simulink model "A3_2_InvKin_testing"  (R2023a)
settings: Solver=VariableStepAuto  StartTime=0.0  StopTime=10.0  RelTol=1e-3
values from neighbouring files (symbols this model uses):
  params = [l2 l3]    [A3_1_init_VorKin.m]    (also in A3_2_init_InvKin.m; init_InvKin.m)
settings Model: Creator=Flo  LastModifiedBy=Flo

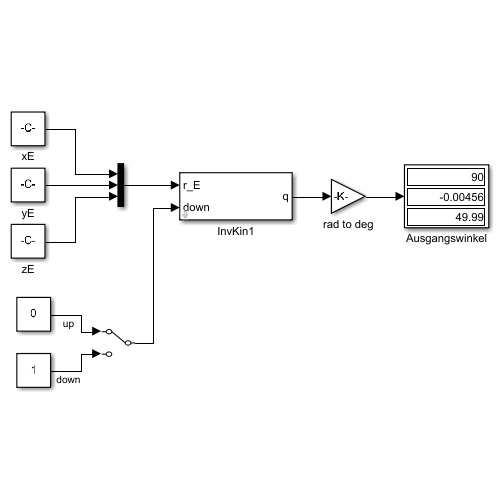
[thumbnail: Simulink's stored preview of the top-level diagram]
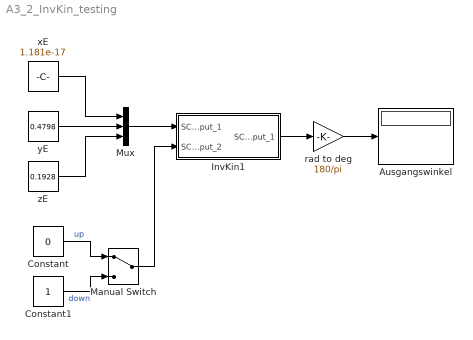
== system A3_2_InvKin_testing ==
  Ausgangswinkel : Display
  Constant : Constant  Value=0
  Constant1 : Constant
  InvKin1 : Subsystem  mask{SC_param_0=params}
      mask prompts: SC_param_0 "params"
      mask Display:
      | port_label('input', 1, 'r_E');
      | port_label('input', 2, 'down');
      | port_label('output', 1, 'q');
  Manual Switch : ManualSwitch
  Mux : Mux  Inputs=3
  rad to deg : Gain  Gain=180/pi
  xE : Constant  Value=1.181e-17
  yE : Constant  Value=0.4798
  zE : Constant  Value=0.1928
  wires:
  zE/1 -> Mux/3
  xE/1 -> Mux/1
  yE/1 -> Mux/2
  Mux/1 -> InvKin1/1(SC_input_1)
  Manual Switch/1 -> InvKin1/2(SC_input_2)
  Constant1/1 -> Manual Switch/2  "down"
  Constant/1 -> Manual Switch/1  "up"
  InvKin1/1(SC_output_1) -> rad to deg/1
  rad to deg/1 -> Ausgangswinkel/1

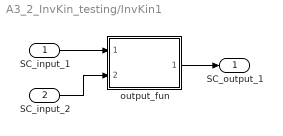
== system A3_2_InvKin_testing/InvKin1 ==
  SC_input_1 : Inport
  SC_input_2 : Inport  Port=2
  output_fun : MATLAB Function  TreatAsAtomicUnit=on
  SC_output_1 : Outport
  wires:
  SC_input_2/1 -> output_fun/2(SC_input_1)
  SC_input_1/1 -> output_fun/1(SC_input_0)
  output_fun/1(SC_output_0) -> SC_output_1/1

== matlab function A3_2_InvKin_testing/InvKin1/output_fun ==
  data: SC_input_0 input size=[3]; SC_output_0 output size=[3]; SC_input_1 input size=[1]; SC_param_0 parameter size=[2]
function SC_output_0  = y_fun(SC_input_0, SC_input_1, SC_param_0)
    SC_output_0 = zeros(3,1);
    SC_output_0(1) = atan2(SC_input_0(3), SC_input_0(1));
    if (SC_input_1(1) == 0)
      s1 = pi / 0.2e1 - atan2(SC_input_0(2), SC_input_0(1) / cos(atan2(SC_input_0(3), SC_input_0(1)))) - asin(SC_param_0(2) * (SC_input_0(1) ^ 2 + SC_input_0(2) ^ 2 + SC_input_0(3) ^ 2) ^ (-0.1e1 / 0.2e1) * sqrt(0.4e1 - (-SC_input_0(1) ^ 2 - SC_input_0(2) ^ 2 - SC_input_0(3) ^ 2 + SC_param_0(1) ^ 2 + SC_param_0(2) ^ 2) ^ 2 / SC_param_0(1) ^ 2 / SC_param_0(2) ^ 2) / 0.2e1);
    else
      s1 = pi / 0.2e1 - atan2(SC_input_0(2), SC_input_0(1) / cos(atan2(SC_input_0(3), SC_input_0(1)))) + asin(SC_param_0(2) * (SC_input_0(1) ^ 2 + SC_input_0(2) ^ 2 + SC_input_0(3) ^ 2) ^ (-0.1e1 / 0.2e1) * sqrt(0.4e1 - (-SC_input_0(1) ^ 2 - SC_input_0(2) ^ 2 - SC_input_0(3) ^ 2 + SC_param_0(1) ^ 2 + SC_param_0(2) ^ 2) ^ 2 / SC_param_0(1) ^ 2 / SC_param_0(2) ^ 2) / 0.2e1);
    end
    SC_output_0(2) = s1;
    if (SC_input_1(1) == 0)
      if (SC_input_1(1) == 0)
        s3 = pi / 0.2e1 - atan2(SC_input_0(2), SC_input_0(1) / cos(atan2(SC_input_0(3), SC_input_0(1)))) - asin(SC_param_0(2) * (SC_input_0(1) ^ 2 + SC_input_0(2) ^ 2 + SC_input_0(3) ^ 2) ^ (-0.1e1 / 0.2e1) * sqrt(0.4e1 - (-SC_input_0(1) ^ 2 - SC_input_0(2) ^ 2 - SC_input_0(3) ^ 2 + SC_param_0(1) ^ 2 + SC_param_0(2) ^ 2) ^ 2 / SC_param_0(1) ^ 2 / SC_param_0(2) ^ 2) / 0.2e1);
      else
        s3 = pi / 0.2e1 - atan2(SC_input_0(2), SC_input_0(1) / cos(atan2(SC_input_0(3), SC_input_0(1)))) + asin(SC_param_0(2) * (SC_input_0(1) ^ 2 + SC_input_0(2) ^ 2 + SC_input_0(3) ^ 2) ^ (-0.1e1 / 0.2e1) * sqrt(0.4e1 - (-SC_input_0(1) ^ 2 - SC_input_0(2) ^ 2 - SC_input_0(3) ^ 2 + SC_param_0(1) ^ 2 + SC_param_0(2) ^ 2) ^ 2 / SC_param_0(1) ^ 2 / SC_param_0(2) ^ 2) / 0.2e1);
      end
      s2 = -pi / 0.2e1 - s3 + acos((-SC_input_0(1) ^ 2 - SC_input_0(2) ^ 2 - SC_input_0(3) ^ 2 + SC_param_0(1) ^ 2 + SC_param_0(2) ^ 2) / SC_param_0(1) / SC_param_0(2) / 0.2e1);
    else
      if (SC_input_1(1) == 0)
        s4 = pi / 0.2e1 - atan2(SC_input_0(2), SC_input_0(1) / cos(atan2(SC_input_0(3), SC_input_0(1)))) - asin(SC_param_0(2) * (SC_input_0(1) ^ 2 + SC_input_0(2) ^ 2 + SC_input_0(3) ^ 2) ^ (-0.1e1 / 0.2e1) * sqrt(0.4e1 - (-SC_input_0(1) ^ 2 - SC_input_0(2) ^ 2 - SC_input_0(3) ^ 2 + SC_param_0(1) ^ 2 + SC_param_0(2) ^ 2) ^ 2 / SC_param_0(1) ^ 2 / SC_param_0(2) ^ 2) / 0.2e1);
      else
        s4 = pi / 0.2e1 - atan2(SC_input_0(2), SC_input_0(1) / cos(atan2(SC_input_0(3), SC_input_0(1)))) + asin(SC_param_0(2) * (SC_input_0(1) ^ 2 + SC_input_0(2) ^ 2 + SC_input_0(3) ^ 2) ^ (-0.1e1 / 0.2e1) * sqrt(0.4e1 - (-SC_input_0(1) ^ 2 - SC_input_0(2) ^ 2 - SC_input_0(3) ^ 2 + SC_param_0(1) ^ 2 + SC_param_0(2) ^ 2) ^ 2 / SC_param_0(1) ^ 2 / SC_param_0(2) ^ 2) / 0.2e1);
      end
      s2 = 0.3e1 / 0.2e1 * pi - s4 - acos((-SC_input_0(1) ^ 2 - SC_input_0(2) ^ 2 - SC_input_0(3) ^ 2 + SC_param_0(1) ^ 2 + SC_param_0(2) ^ 2) / SC_param_0(1) / SC_param_0(2) / 0.2e1);
    end
    SC_output_0(3) = s2;
end
